simulink model "Template"  (R2021b)
settings: Solver=VariableStepAuto  StartTime=0.0  StopTime=48  RelTol=1e-3
undefined symbols (not defined in the file or in its folder): f650
libraries: simulink x32, slpidlib x1
settings Model: Creator=Admin  LastModifiedBy=Admin
settings SolverCC: AlgebraicLoopSolver=TrustRegion
settings DebuggingCC: SFMachineParentedDataDiag=warning

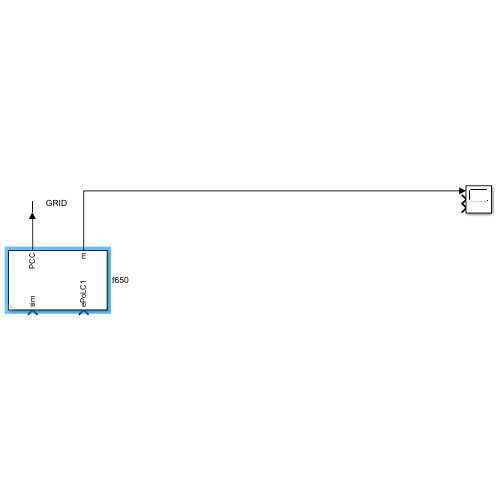
[thumbnail: Simulink's stored preview of the top-level diagram]
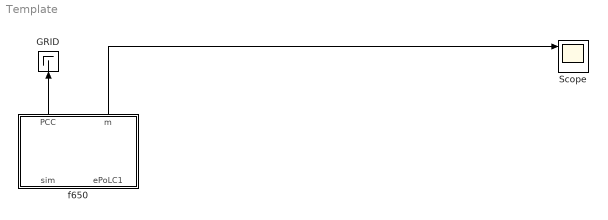
== system Template ==
  GRID : Terminator
  Scope : Scope  NumInputPorts=3
  f650 : Subsystem  mask(Prosumer){sPoLC1sel=External, sPoLC2sel=Disabled, sPoLC3sel=Disabled, sPoLC4sel=Disabled, sPoLC5sel=Disabled, sPoLC6sel=Disabled, sPoLC7sel=Disabled, sPoLC8sel=Disabled, sPoLC9sel=Disabled, sPoLC10sel=Disabled, sPoLC11sel=Disabled, sPoLC12sel=Disabled, sPoLC13sel=Disabled, sPoLC14sel=Disabled, sPoLC15sel=Disabled, sPoLC16sel=Disabled}
      mask prompts: sPoLC1sel "PoLC #1 type"; sPoLC2sel "PoLC #2 type"; sPoLC3sel "PoLC #3 type"; sPoLC4sel "PoLC #4 type"; sPoLC5sel "PoLC #5 type"; sPoLC6sel "PoLC #6 type"; sPoLC7sel "PoLC #7 type"; sPoLC8sel "PoLC #8 type"; sPoLC9sel "PoLC #9 type"; sPoLC10sel "PoLC #10 type"; sPoLC11sel "PoLC #11 type"; sPoLC12sel "PoLC #12 type"; sPoLC13sel "PoLC #13 type"; sPoLC14sel "PoLC #14 type"; sPoLC15sel "PoLC #15 type"; sPoLC16sel "PoLC #16 type"
      mask help:
      | Simplified model of electrical prosumer technological system.
      |
      | V0.1.0
      mask init:
      | % link local generation variables
      | tblk = Simulink.findBlocks(gcb,'Name','base');
      | for i=1:length(tblk)
      |     val = strrep(getfullname(tblk(i)),join([gcs,'/'],''),'');
      |     val = strrep(val,join(['/','base'],''),'');
      |     val = strrep(val,'lPoLC','PoLC');
      |     val = strrep(val,'DEVICES/','');
      |     val = strrep(val,'CONTROLLERS/','');
      |     val = strrep(val,'/','.');
      |     set_param(tblk(i),'OutValues',join([val,'.','l'],''));
      |     set_param(tblk(i),'tsamp',join([val,'.','ST'],''));
      | end
      | 
      | sblk = Simulink.findBlocks(gcb,'Name','noise');
      | for i=1:length(sblk)
      |     val = strrep(getfullname(sblk(i)),join([gcs,'/'],''),'');
      |     val = strrep(val,join(['/','noise'],''),'');
      |     val = strrep(val,'lPoLC','PoLC');
      |     val = strrep(val,'DEVICES/','');
      |     val = strrep(val,'CONTROLLERS/','');
      |     val = strrep(val,'/','.');
      |     set_param(sblk(i),'Cov',join([val,'.','Noise'],''));
      |     set_param(sblk(i),'Ts',join([val,'.','NoiseST'],''));
      |     set_param(sblk(i),'seed',join([val,'.','NoiseSD'],''));
      | end
      mask TypeOptions sPoLC1sel: Disabled | Internal | External
      mask Callback sPoLC1sel: prsmr_functions('1',gcs,gcb);
      mask TypeOptions sPoLC2sel: Disabled | Internal | External
      mask Callback sPoLC2sel: prsmr_functions('2',gcs,gcb)
      mask TypeOptions sPoLC3sel: Disabled | Internal | External
      mask Callback sPoLC3sel: prsmr_functions('3',gcs,gcb)
      mask TypeOptions sPoLC4sel: Disabled | Internal | External
      mask Callback sPoLC4sel: prsmr_functions('4',gcs,gcb)
      mask TypeOptions sPoLC5sel: Disabled | Internal | External
      mask Callback sPoLC5sel: prsmr_functions('5',gcs,gcb)
      mask TypeOptions sPoLC6sel: Disabled | Internal | External
      mask Callback sPoLC6sel: prsmr_functions('6',gcs,gcb)
      mask TypeOptions sPoLC7sel: Disabled | Internal | External
      mask Callback sPoLC7sel: prsmr_functions('7',gcs,gcb)
      mask TypeOptions sPoLC8sel: Disabled | Internal | External
      mask Callback sPoLC8sel: prsmr_functions('8',gcs,gcb)
      mask TypeOptions sPoLC9sel: Disabled | Internal | External
      mask Callback sPoLC9sel: prsmr_functions('9',gcs,gcb)
      mask TypeOptions sPoLC10sel: Disabled | Internal | External
      mask Callback sPoLC10sel: prsmr_functions('10',gcs,gcb)
      mask TypeOptions sPoLC11sel: Disabled | Internal | External
      mask Callback sPoLC11sel: prsmr_functions('11',gcs,gcb)
      mask TypeOptions sPoLC12sel: Disabled | Internal | External
      mask Callback sPoLC12sel: prsmr_functions('12',gcs,gcb)
      mask TypeOptions sPoLC13sel: Disabled | Internal | External
      mask Callback sPoLC13sel: prsmr_functions('13',gcs,gcb)
      mask TypeOptions sPoLC14sel: Disabled | Internal | External
      mask Callback sPoLC14sel: prsmr_functions('14',gcs,gcb)
      mask TypeOptions sPoLC15sel: Disabled | Internal | External
      mask Callback sPoLC15sel: prsmr_functions('15',gcs,gcb)
      mask TypeOptions sPoLC16sel: Disabled | Internal | External
      mask Callback sPoLC16sel: prsmr_functions('16',gcs,gcb)
  wires:
  f650/2(m) -> Scope/1
  f650/1(PCC) -> GRID/1

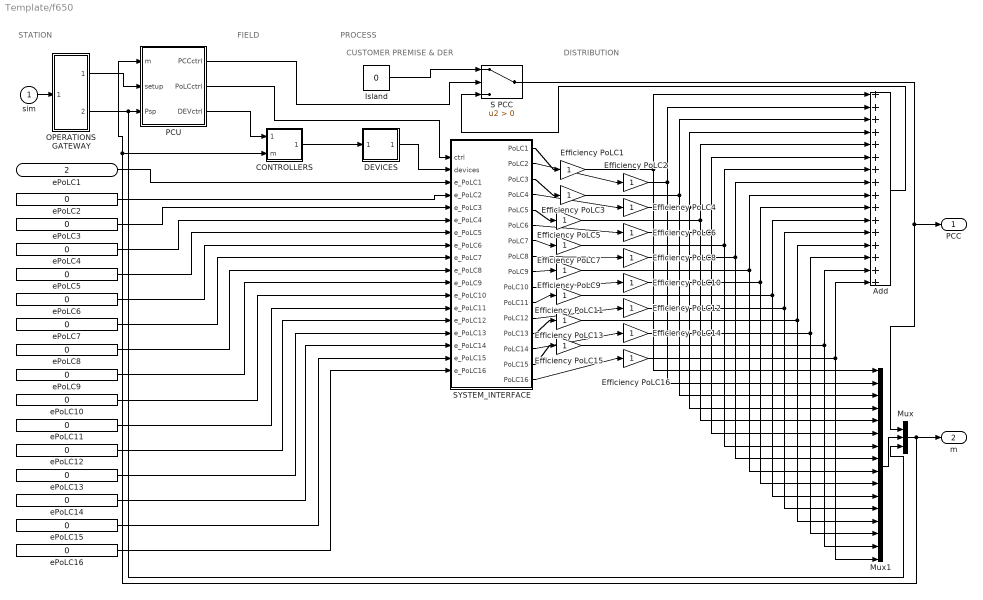
== system Template/f650 ==
  note: PROCESS
  note: STATION
  note: FIELD
  note: DISTRIBUTION
  note: CUSTOMER PREMISE & DER
  sim : Inport
  ePoLC1 : Inport  Port=2
  Add : Sum  Inputs=16
  CONTROLLERS : Subsystem
  DEVICES : Subsystem
  Efficiency PoLC{1..16} (16 alike) : Gain  ParamMin=[0]  ParamMax=[1]
  Island : Constant  Value=0
  Mux : Mux  Inputs=3
  Mux1 : Mux  Inputs=16
  OPERATIONS GATEWAY : Subsystem
  PCU : Subsystem
  S PCC : Switch  Criteria=u2 > Threshold
  SYSTEM_INTERFACE : Subsystem
  ePoLC{2..16} (15 alike) : Constant  Value=0
  PCC : Outport  VectorParamsAs1DForOutWhenUnconnected=off
  m : Outport  Port=2  VectorParamsAs1DForOutWhenUnconnected=off
  wires:
  PCU/1(PCCctrl) -> S PCC/2
  Mux1/1 -> Mux/2
  Island/1 -> S PCC/1
  Mux/1 -> CONTROLLERS/2(m), PCU/1(m), m/1
  S PCC/1 -> Mux/1, PCC/1
  Add/1 -> S PCC/3
  SYSTEM_INTERFACE/2(PoLC2) -> Efficiency PoLC2/1
  SYSTEM_INTERFACE/4(PoLC4) -> Efficiency PoLC4/1
  SYSTEM_INTERFACE/8(PoLC8) -> Efficiency PoLC8/1
  SYSTEM_INTERFACE/5(PoLC5) -> Efficiency PoLC5/1
  SYSTEM_INTERFACE/12(PoLC12) -> Efficiency PoLC12/1
  SYSTEM_INTERFACE/15(PoLC15) -> Efficiency PoLC15/1
  SYSTEM_INTERFACE/6(PoLC6) -> Efficiency PoLC6/1
  SYSTEM_INTERFACE/13(PoLC13) -> Efficiency PoLC13/1
  SYSTEM_INTERFACE/10(PoLC10) -> Efficiency PoLC10/1
  SYSTEM_INTERFACE/3(PoLC3) -> Efficiency PoLC3/1
  SYSTEM_INTERFACE/16(PoLC16) -> Efficiency PoLC16/1
  SYSTEM_INTERFACE/1(PoLC1) -> Efficiency PoLC1/1
  SYSTEM_INTERFACE/11(PoLC11) -> Efficiency PoLC11/1
  SYSTEM_INTERFACE/9(PoLC9) -> Efficiency PoLC9/1
  SYSTEM_INTERFACE/7(PoLC7) -> Efficiency PoLC7/1
  SYSTEM_INTERFACE/14(PoLC14) -> Efficiency PoLC14/1
  ePoLC1/1 -> SYSTEM_INTERFACE/3(e_PoLC1)
  ePoLC2/1 -> SYSTEM_INTERFACE/4(e_PoLC2)
  ePoLC3/1 -> SYSTEM_INTERFACE/5(e_PoLC3)
  ePoLC4/1 -> SYSTEM_INTERFACE/6(e_PoLC4)
  ePoLC5/1 -> SYSTEM_INTERFACE/7(e_PoLC5)
  ePoLC6/1 -> SYSTEM_INTERFACE/8(e_PoLC6)
  ePoLC7/1 -> SYSTEM_INTERFACE/9(e_PoLC7)
  ePoLC8/1 -> SYSTEM_INTERFACE/10(e_PoLC8)
  ePoLC9/1 -> SYSTEM_INTERFACE/11(e_PoLC9)
  ePoLC10/1 -> SYSTEM_INTERFACE/12(e_PoLC10)
  ePoLC11/1 -> SYSTEM_INTERFACE/13(e_PoLC11)
  ePoLC12/1 -> SYSTEM_INTERFACE/14(e_PoLC12)
  ePoLC13/1 -> SYSTEM_INTERFACE/15(e_PoLC13)
  ePoLC14/1 -> SYSTEM_INTERFACE/16(e_PoLC14)
  ePoLC15/1 -> SYSTEM_INTERFACE/17(e_PoLC15)
  ePoLC16/1 -> SYSTEM_INTERFACE/18(e_PoLC16)
  PCU/2(PoLCctrl) -> SYSTEM_INTERFACE/1(ctrl)
  CONTROLLERS/1(dev) -> DEVICES/1(ctrl)
  OPERATIONS GATEWAY/1(setup) -> PCU/2(setup)
  OPERATIONS GATEWAY/2(Psp) -> Mux/3, PCU/3(Psp)
  sim/1 -> OPERATIONS GATEWAY/1(sim)
  PCU/3(DEVctrl) -> CONTROLLERS/1(ctrl)
  DEVICES/1(dev) -> SYSTEM_INTERFACE/2(devices)
  Efficiency PoLC1/1 -> Add/1, Mux1/1
  Efficiency PoLC2/1 -> Add/2, Mux1/2
  Efficiency PoLC3/1 -> Add/3, Mux1/3
  Efficiency PoLC4/1 -> Add/4, Mux1/4
  Efficiency PoLC5/1 -> Add/5, Mux1/5
  Efficiency PoLC6/1 -> Add/6, Mux1/6
  Efficiency PoLC7/1 -> Add/7, Mux1/7
  Efficiency PoLC8/1 -> Add/8, Mux1/8
  Efficiency PoLC9/1 -> Add/9, Mux1/9
  Efficiency PoLC10/1 -> Mux1/10, Add/10
  Efficiency PoLC11/1 -> Add/11, Mux1/11
  Efficiency PoLC12/1 -> Add/12, Mux1/12
  Efficiency PoLC13/1 -> Add/13, Mux1/13
  Efficiency PoLC14/1 -> Add/14, Mux1/14
  Efficiency PoLC15/1 -> Mux1/15, Add/15
  Efficiency PoLC16/1 -> Add/16, Mux1/16

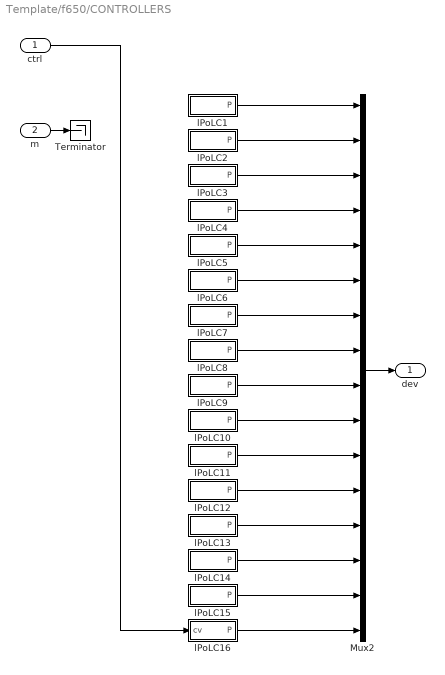
== system Template/f650/CONTROLLERS ==
  ctrl : Inport
  m : Inport  Port=2
  Mux2 : Mux  Inputs=16
  Terminator : Terminator
  lPoLC1 : Subsystem  TreatAsAtomicUnit=on
  lPoLC10 : Subsystem  TreatAsAtomicUnit=on
  lPoLC11 : Subsystem  TreatAsAtomicUnit=on
  lPoLC12 : Subsystem  TreatAsAtomicUnit=on
  lPoLC13 : Subsystem  TreatAsAtomicUnit=on
  lPoLC14 : Subsystem  TreatAsAtomicUnit=on
  lPoLC15 : Subsystem  TreatAsAtomicUnit=on
  lPoLC16 : Subsystem  TreatAsAtomicUnit=on
  lPoLC2 : Subsystem  TreatAsAtomicUnit=on
  lPoLC3 : Subsystem  TreatAsAtomicUnit=on
  lPoLC4 : Subsystem  TreatAsAtomicUnit=on
  lPoLC5 : Subsystem  TreatAsAtomicUnit=on
  lPoLC6 : Subsystem  TreatAsAtomicUnit=on
  lPoLC7 : Subsystem  TreatAsAtomicUnit=on
  lPoLC8 : Subsystem  TreatAsAtomicUnit=on
  lPoLC9 : Subsystem  TreatAsAtomicUnit=on
  dev : Outport  VectorParamsAs1DForOutWhenUnconnected=off
  wires:
  Mux2/1 -> dev/1
  lPoLC1/1(P) -> Mux2/1
  lPoLC2/1(P) -> Mux2/2
  lPoLC16/1(P) -> Mux2/16
  lPoLC3/1(P) -> Mux2/3
  lPoLC4/1(P) -> Mux2/4
  lPoLC5/1(P) -> Mux2/5
  lPoLC6/1(P) -> Mux2/6
  lPoLC7/1(P) -> Mux2/7
  lPoLC8/1(P) -> Mux2/8
  lPoLC9/1(P) -> Mux2/9
  lPoLC10/1(P) -> Mux2/10
  lPoLC11/1(P) -> Mux2/11
  lPoLC12/1(P) -> Mux2/12
  lPoLC13/1(P) -> Mux2/13
  lPoLC14/1(P) -> Mux2/14
  lPoLC15/1(P) -> Mux2/15
  ctrl/1 -> lPoLC16/1(cv)
  m/1 -> Terminator/1

== system Template/f650/DEVICES ==
  ctrl : Inport
  dev : Outport  VectorParamsAs1DForOutWhenUnconnected=off
  wires:
  ctrl/1 -> dev/1

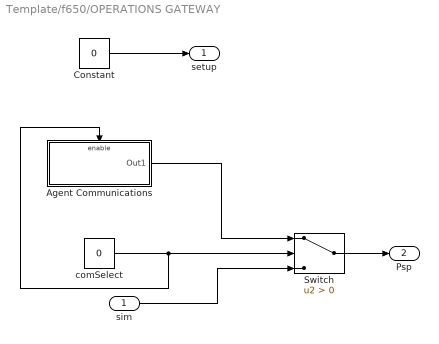
== system Template/f650/OPERATIONS GATEWAY ==
  sim : Inport
  Agent Communications : Subsystem  TreatAsAtomicUnit=on
  Constant : Constant  Value=0
  Switch : Switch  Criteria=u2 > Threshold
  comSelect : Constant  Value=0
  setup : Outport  VectorParamsAs1DForOutWhenUnconnected=off
  Psp : Outport  Port=2  VectorParamsAs1DForOutWhenUnconnected=off
  wires:
  Constant/1 -> setup/1
  sim/1 -> Switch/3
  Switch/1 -> Psp/1
  Agent Communications/1(Out1) -> Switch/1
  comSelect/1 -> Switch/2, Agent Communications/Enable

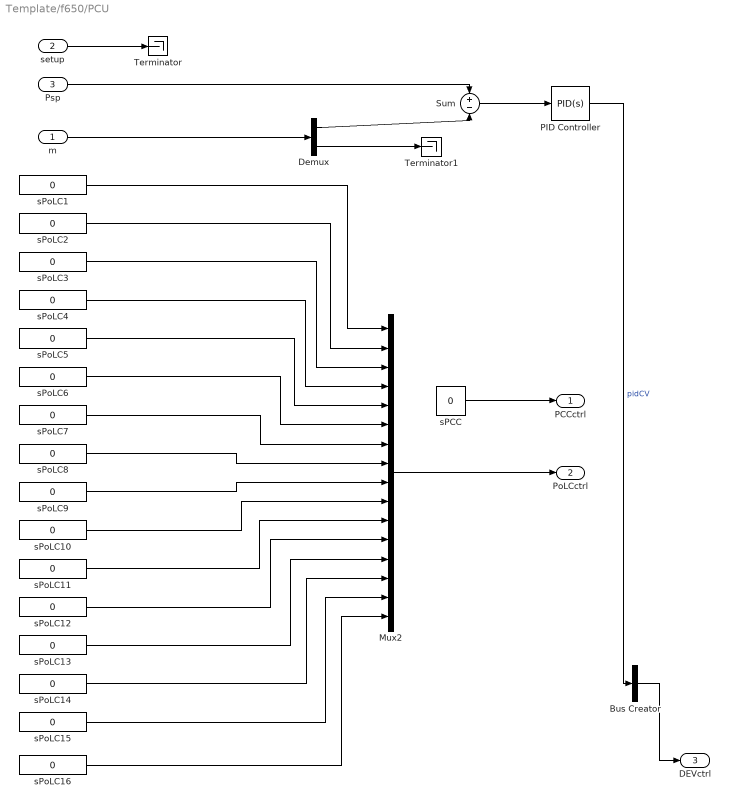
== system Template/f650/PCU ==
  m : Inport
  setup : Inport  Port=2
  Psp : Inport  Port=3
  Bus Creator : BusCreator  Inputs=1
  Demux : Demux  Outputs=[1 -1]
  Mux2 : Mux  Inputs=16
  PID Controller : slpidlib/PID Controller  Controller=PID  Form=Parallel  TimeDomain=Continuous-time  UseExternalTs=off  SampleTime=-1  IntegratorMethod=Forward Euler  FilterMethod=Forward Euler  ControllerParametersSource=internal  P=80  I=20  D=10  UseFilter=on  N=100  TunerSelectOption=Transfer Function Based (PID Tuner App)  InitialConditionSource=internal  InitialConditionForIntegrator=0  InitialConditionForFilter=0  DifferentiatorICPrevScaledInput=0  ExternalReset=none  TrackingMode=off  Kt=1  LimitOutput=off  SatLimitsSource=internal  UpperSaturationLimit=inf  LowerSaturationLimit=-inf  LinearizeAsGain=on  AntiWindupMode=none  Kb=1  POutMin=[]  POutMax=[]  IOutMin=[]  IOutMax=[]  DOutMin=[]  DOutMax=[]  NOutMin=[]  NOutMax=[]  SumOutMin=[]  SumOutMax=[]  SaturationOutMin=[]  SaturationOutMax=[]  PParamMin=[]  PParamMax=[]  IParamMin=[]  IParamMax=[]  DParamMin=[]  DParamMax=[]  NParamMin=[]  NParamMax=[]  KbParamMin=[]  KbParamMax=[]  KtParamMin=[]  KtParamMax=[]  KbOutMin=[]  KbOutMax=[]  KtOutMin=[]  KtOutMax=[]  IntegratorOutMin=[]  IntegratorOutMax=[]  FilterOutMin=[]  FilterOutMax=[]  SumI1OutMin=[]  SumI1OutMax=[]  SumI2OutMin=[]  SumI2OutMax=[]  SumI3OutMin=[]  SumI3OutMax=[]  SumI4OutMin=[]  SumI4OutMax=[]  SumDOutMin=[]  SumDOutMax=[]  DifferentiatorOutMin=[]  DifferentiatorOutMax=[]  FilterDiffOutCoefMin=[]  FilterDiffOutCoefMax=[]  ReciprocalOutMin=[]  ReciprocalOutMax=[]  SumDenOutMin=[]  SumDenOutMax=[]  SumNumOutMin=[]  SumNumOutMax=[]  DivideOutMin=[]  DivideOutMax=[]  UdiffTsProdOutMin=[]  UdiffTsProdOutMax=[]  NTsProdOutMin=[]  NTsProdOutMax=[]  UintegralTsProdOutMin=[]  UintegralTsProdOutMax=[]  UngainTsProdOutMin=[]  UngainTsProdOutMax=[]  IntegratorContinuousStateAttributes=''  IntegratorStateMustResolveToSignalObject=off  IntegratorRTWStateStorageClass=Auto  FilterContinuousStateAttributes=''  FilterStateMustResolveToSignalObject=off  FilterRTWStateStorageClass=Auto  ParallelPVariant=InternalParameters  IdealPVariant=Disabled  IVariant=InternalParameters  DVariant=InternalParameters  IntegratorVariant=Continuous  SatVariant=Disabled  AWVariant=Passthrough  PCopyVariant=Disabled  TRVariant=Disabled  FdbkBlocksVariant=Forward  IdealPFdbkVariant=Disabled  SatFdbkVariant=Disabled  DerivativeFilterVariant=ContFilter  NVariant=InternalParameters  NCopyVariant=Disabled  FilterICVariant=InternalICsFilter  IntegratorICVariant=InternalICs  ExternalResetVariant=Disabled  TRSumVariant=Passthrough  SumFdbkVariant=Disabled  SumVariant=Sum_PID  TsampFilterVariant=InternalTs  TsampNgainVariant=Passthrough  TsampIntegralVariant=Passthrough  ExternalSaturationOutDataTypeStr=Inherit: Same as second input
  Sum : Sum  Inputs=+-
  Terminator : Terminator
  Terminator1 : Terminator
  sPCC : Constant  Value=0
  sPoLC{1..16} (16 alike) : Constant  Value=0
  PCCctrl : Outport  VectorParamsAs1DForOutWhenUnconnected=off
  PoLCctrl : Outport  Port=2  VectorParamsAs1DForOutWhenUnconnected=off
  DEVctrl : Outport  Port=3  VectorParamsAs1DForOutWhenUnconnected=off
  wires:
  sPoLC8/1 -> Mux2/8
  sPoLC11/1 -> Mux2/11
  sPoLC4/1 -> Mux2/4
  sPoLC16/1 -> Mux2/16
  sPoLC14/1 -> Mux2/14
  sPoLC10/1 -> Mux2/10
  sPoLC12/1 -> Mux2/12
  sPoLC1/1 -> Mux2/1
  sPoLC15/1 -> Mux2/15
  sPoLC6/1 -> Mux2/6
  sPoLC13/1 -> Mux2/13
  sPoLC7/1 -> Mux2/7
  sPoLC9/1 -> Mux2/9
  sPoLC2/1 -> Mux2/2
  sPoLC3/1 -> Mux2/3
  sPoLC5/1 -> Mux2/5
  Mux2/1 -> PoLCctrl/1
  sPCC/1 -> PCCctrl/1
  setup/1 -> Terminator/1
  Psp/1 -> Sum/1
  Bus Creator/1 -> DEVctrl/1
  m/1 -> Demux/1
  Demux/1 -> Sum/2
  Sum/1 -> PID Controller/1
  PID Controller/1 -> Bus Creator/1  "pidCV"
  Demux/2 -> Terminator1/1

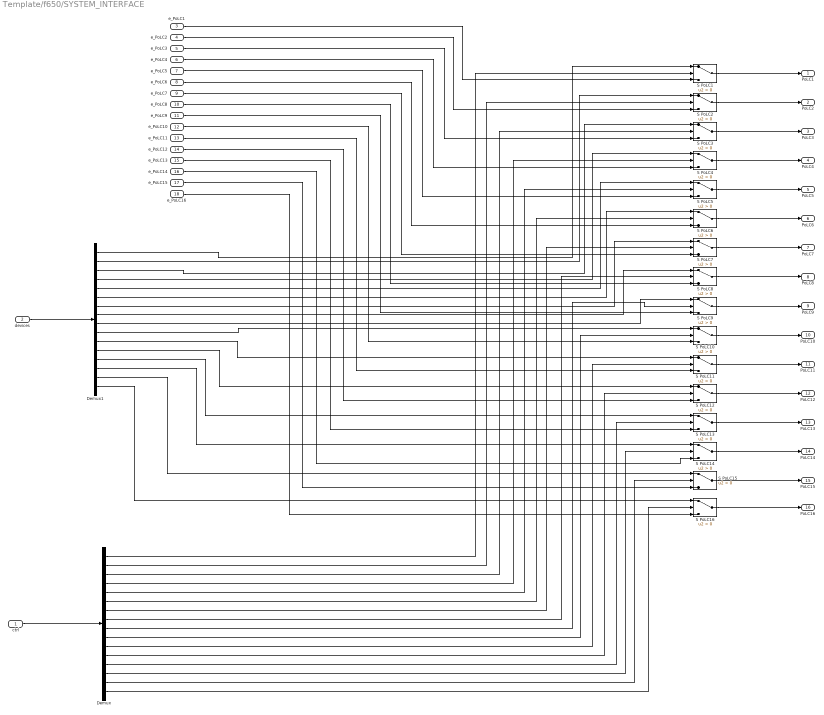
== system Template/f650/SYSTEM_INTERFACE ==
  ctrl : Inport
  devices : Inport  Port=2
  e_PoLC1 : Inport  Port=3
  e_PoLC2 : Inport  Port=4
  e_PoLC3 : Inport  Port=5
  e_PoLC4 : Inport  Port=6
  e_PoLC5 : Inport  Port=7
  e_PoLC6 : Inport  Port=8
  e_PoLC7 : Inport  Port=9
  e_PoLC8 : Inport  Port=10
  e_PoLC9 : Inport  Port=11
  e_PoLC10 : Inport  Port=12
  e_PoLC11 : Inport  Port=13
  e_PoLC12 : Inport  Port=14
  e_PoLC13 : Inport  Port=15
  e_PoLC14 : Inport  Port=16
  e_PoLC15 : Inport  Port=17
  e_PoLC16 : Inport  Port=18
  Demux : Demux  Outputs=16
  Demux1 : Demux  Outputs=16
  S PoLC{1..16} (16 alike) : Switch  Criteria=u2 > Threshold
  PoLC1 : Outport  VectorParamsAs1DForOutWhenUnconnected=off
  PoLC2 : Outport  Port=2  VectorParamsAs1DForOutWhenUnconnected=off
  PoLC3 : Outport  Port=3  VectorParamsAs1DForOutWhenUnconnected=off
  PoLC4 : Outport  Port=4  VectorParamsAs1DForOutWhenUnconnected=off
  PoLC5 : Outport  Port=5  VectorParamsAs1DForOutWhenUnconnected=off
  PoLC6 : Outport  Port=6  VectorParamsAs1DForOutWhenUnconnected=off
  PoLC7 : Outport  Port=7  VectorParamsAs1DForOutWhenUnconnected=off
  PoLC8 : Outport  Port=8  VectorParamsAs1DForOutWhenUnconnected=off
  PoLC9 : Outport  Port=9  VectorParamsAs1DForOutWhenUnconnected=off
  PoLC10 : Outport  Port=10  VectorParamsAs1DForOutWhenUnconnected=off
  PoLC11 : Outport  Port=11  VectorParamsAs1DForOutWhenUnconnected=off
  PoLC12 : Outport  Port=12  VectorParamsAs1DForOutWhenUnconnected=off
  PoLC13 : Outport  Port=13  VectorParamsAs1DForOutWhenUnconnected=off
  PoLC14 : Outport  Port=14  VectorParamsAs1DForOutWhenUnconnected=off
  PoLC15 : Outport  Port=15  VectorParamsAs1DForOutWhenUnconnected=off
  PoLC16 : Outport  Port=16  VectorParamsAs1DForOutWhenUnconnected=off
  wires:
  S PoLC9/1 -> PoLC9/1
  e_PoLC4/1 -> S PoLC4/3
  e_PoLC11/1 -> S PoLC11/3
  S PoLC16/1 -> PoLC16/1
  e_PoLC8/1 -> S PoLC8/3
  S PoLC6/1 -> PoLC6/1
  e_PoLC7/1 -> S PoLC7/3
  S PoLC13/1 -> PoLC13/1
  e_PoLC5/1 -> S PoLC5/3
  S PoLC10/1 -> PoLC10/1
  e_PoLC9/1 -> S PoLC9/3
  e_PoLC12/1 -> S PoLC12/3
  e_PoLC6/1 -> S PoLC6/3
  S PoLC15/1 -> PoLC15/1
  S PoLC1/1 -> PoLC1/1
  S PoLC12/1 -> PoLC12/1
  S PoLC11/1 -> PoLC11/1
  e_PoLC14/1 -> S PoLC14/3
  e_PoLC10/1 -> S PoLC10/3
  S PoLC5/1 -> PoLC5/1
  e_PoLC1/1 -> S PoLC1/3
  e_PoLC15/1 -> S PoLC15/3
  e_PoLC16/1 -> S PoLC16/3
  S PoLC7/1 -> PoLC7/1
  e_PoLC3/1 -> S PoLC3/3
  e_PoLC13/1 -> S PoLC13/3
  S PoLC8/1 -> PoLC8/1
  e_PoLC2/1 -> S PoLC2/3
  S PoLC4/1 -> PoLC4/1
  S PoLC2/1 -> PoLC2/1
  S PoLC14/1 -> PoLC14/1
  S PoLC3/1 -> PoLC3/1
  ctrl/1 -> Demux/1
  Demux/1 -> S PoLC1/2
  Demux/2 -> S PoLC2/2
  Demux/3 -> S PoLC3/2
  Demux/4 -> S PoLC4/2
  Demux/5 -> S PoLC5/2
  Demux/6 -> S PoLC6/2
  Demux/7 -> S PoLC7/2
  Demux/8 -> S PoLC8/2
  Demux/9 -> S PoLC9/2
  Demux/10 -> S PoLC10/2
  Demux/11 -> S PoLC11/2
  Demux/12 -> S PoLC12/2
  Demux/13 -> S PoLC13/2
  Demux/14 -> S PoLC14/2
  Demux/15 -> S PoLC15/2
  Demux/16 -> S PoLC16/2
  devices/1 -> Demux1/1
  Demux1/1 -> S PoLC1/1
  Demux1/2 -> S PoLC2/1
  Demux1/3 -> S PoLC3/1
  Demux1/4 -> S PoLC4/1
  Demux1/5 -> S PoLC5/1
  Demux1/6 -> S PoLC6/1
  Demux1/7 -> S PoLC7/1
  Demux1/8 -> S PoLC8/1
  Demux1/9 -> S PoLC9/1
  Demux1/10 -> S PoLC10/1
  Demux1/11 -> S PoLC11/1
  Demux1/12 -> S PoLC12/1
  Demux1/13 -> S PoLC13/1
  Demux1/14 -> S PoLC14/1
  Demux1/15 -> S PoLC15/1
  Demux1/16 -> S PoLC16/1

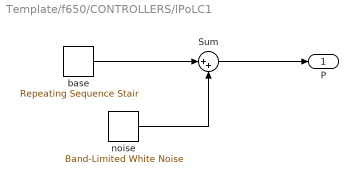
== system Template/f650/CONTROLLERS/lPoLC1 ==
  Sum : Sum  Inputs=|++
  base : simulink/Sources/Repeating Sequence Stair  OutValues=f650.PoLC1.l  tsamp=f650.PoLC1.ST  OutMin=[]  OutMax=[]  OutDataTypeStr=double  OutputDataTypeScalingMode=double  OutDataType=fixdt(0,8)  ConRadixGroup=Best Precision: Vector-wise  OutScaling=2^-12
  noise : simulink/Sources/Band-Limited White Noise  Cov=f650.PoLC1.Noise  Ts=f650.PoLC1.NoiseST  seed=f650.PoLC1.NoiseSD
  P : Outport  VectorParamsAs1DForOutWhenUnconnected=off
  wires:
  Sum/1 -> P/1
  noise/1 -> Sum/2
  base/1 -> Sum/1

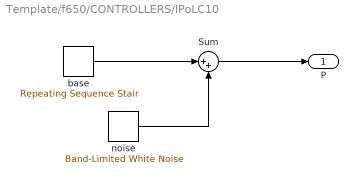
== system Template/f650/CONTROLLERS/lPoLC10 ==
  Sum : Sum  Inputs=|++
  base : simulink/Sources/Repeating Sequence Stair  OutValues=f650.PoLC10.l  tsamp=f650.PoLC10.ST  OutMin=[]  OutMax=[]  OutDataTypeStr=double  OutputDataTypeScalingMode=double  OutDataType=fixdt(0,8)  ConRadixGroup=Best Precision: Vector-wise  OutScaling=2^-12
  noise : simulink/Sources/Band-Limited White Noise  Cov=f650.PoLC10.Noise  Ts=f650.PoLC10.NoiseST  seed=f650.PoLC10.NoiseSD
  P : Outport  VectorParamsAs1DForOutWhenUnconnected=off
  wires:
  Sum/1 -> P/1
  noise/1 -> Sum/2
  base/1 -> Sum/1

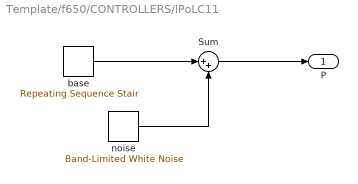
== system Template/f650/CONTROLLERS/lPoLC11 ==
  Sum : Sum  Inputs=|++
  base : simulink/Sources/Repeating Sequence Stair  OutValues=f650.PoLC11.l  tsamp=f650.PoLC11.ST  OutMin=[]  OutMax=[]  OutDataTypeStr=double  OutputDataTypeScalingMode=double  OutDataType=fixdt(0,8)  ConRadixGroup=Best Precision: Vector-wise  OutScaling=2^-12
  noise : simulink/Sources/Band-Limited White Noise  Cov=f650.PoLC11.Noise  Ts=f650.PoLC11.NoiseST  seed=f650.PoLC11.NoiseSD
  P : Outport  VectorParamsAs1DForOutWhenUnconnected=off
  wires:
  Sum/1 -> P/1
  noise/1 -> Sum/2
  base/1 -> Sum/1

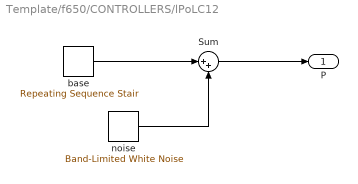
== system Template/f650/CONTROLLERS/lPoLC12 ==
  Sum : Sum  Inputs=|++
  base : simulink/Sources/Repeating Sequence Stair  OutValues=f650.PoLC12.l  tsamp=f650.PoLC12.ST  OutMin=[]  OutMax=[]  OutDataTypeStr=double  OutputDataTypeScalingMode=double  OutDataType=fixdt(0,8)  ConRadixGroup=Best Precision: Vector-wise  OutScaling=2^-12
  noise : simulink/Sources/Band-Limited White Noise  Cov=f650.PoLC12.Noise  Ts=f650.PoLC12.NoiseST  seed=f650.PoLC12.NoiseSD
  P : Outport  VectorParamsAs1DForOutWhenUnconnected=off
  wires:
  Sum/1 -> P/1
  noise/1 -> Sum/2
  base/1 -> Sum/1

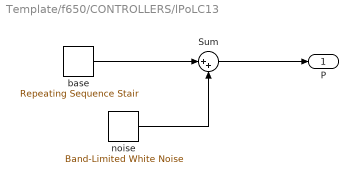
== system Template/f650/CONTROLLERS/lPoLC13 ==
  Sum : Sum  Inputs=|++
  base : simulink/Sources/Repeating Sequence Stair  OutValues=f650.PoLC13.l  tsamp=f650.PoLC13.ST  OutMin=[]  OutMax=[]  OutDataTypeStr=double  OutputDataTypeScalingMode=double  OutDataType=fixdt(0,8)  ConRadixGroup=Best Precision: Vector-wise  OutScaling=2^-12
  noise : simulink/Sources/Band-Limited White Noise  Cov=f650.PoLC13.Noise  Ts=f650.PoLC13.NoiseST  seed=f650.PoLC13.NoiseSD
  P : Outport  VectorParamsAs1DForOutWhenUnconnected=off
  wires:
  Sum/1 -> P/1
  noise/1 -> Sum/2
  base/1 -> Sum/1

== system Template/f650/CONTROLLERS/lPoLC14 ==
  Sum : Sum  Inputs=|++
  base : simulink/Sources/Repeating Sequence Stair  OutValues=f650.PoLC14.l  tsamp=f650.PoLC14.ST  OutMin=[]  OutMax=[]  OutDataTypeStr=double  OutputDataTypeScalingMode=double  OutDataType=fixdt(0,8)  ConRadixGroup=Best Precision: Vector-wise  OutScaling=2^-12
  noise : simulink/Sources/Band-Limited White Noise  Cov=f650.PoLC14.Noise  Ts=f650.PoLC14.NoiseST  seed=f650.PoLC14.NoiseSD
  P : Outport  VectorParamsAs1DForOutWhenUnconnected=off
  wires:
  Sum/1 -> P/1
  noise/1 -> Sum/2
  base/1 -> Sum/1

== system Template/f650/CONTROLLERS/lPoLC15 ==
  Sum : Sum  Inputs=|++
  base : simulink/Sources/Repeating Sequence Stair  OutValues=f650.PoLC15.l  tsamp=f650.PoLC15.ST  OutMin=[]  OutMax=[]  OutDataTypeStr=double  OutputDataTypeScalingMode=double  OutDataType=fixdt(0,8)  ConRadixGroup=Best Precision: Vector-wise  OutScaling=2^-12
  noise : simulink/Sources/Band-Limited White Noise  Cov=f650.PoLC15.Noise  Ts=f650.PoLC15.NoiseST  seed=f650.PoLC15.NoiseSD
  P : Outport  VectorParamsAs1DForOutWhenUnconnected=off
  wires:
  Sum/1 -> P/1
  noise/1 -> Sum/2
  base/1 -> Sum/1

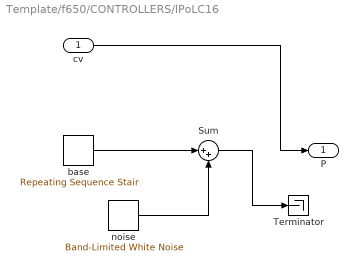
== system Template/f650/CONTROLLERS/lPoLC16 ==
  cv : Inport
  Sum : Sum  Inputs=|++
  Terminator : Terminator
  base : simulink/Sources/Repeating Sequence Stair  OutValues=f650.PoLC16.l  tsamp=f650.PoLC16.ST  OutMin=[]  OutMax=[]  OutDataTypeStr=double  OutputDataTypeScalingMode=double  OutDataType=fixdt(0,8)  ConRadixGroup=Best Precision: Vector-wise  OutScaling=2^-12
  noise : simulink/Sources/Band-Limited White Noise  Cov=f650.PoLC16.Noise  Ts=f650.PoLC16.NoiseST  seed=f650.PoLC16.NoiseSD
  P : Outport  VectorParamsAs1DForOutWhenUnconnected=off
  wires:
  Sum/1 -> Terminator/1
  noise/1 -> Sum/2
  base/1 -> Sum/1
  cv/1 -> P/1

== system Template/f650/CONTROLLERS/lPoLC2 ==
  Sum : Sum  Inputs=|++
  base : simulink/Sources/Repeating Sequence Stair  OutValues=f650.PoLC2.l  tsamp=f650.PoLC2.ST  OutMin=[]  OutMax=[]  OutDataTypeStr=double  OutputDataTypeScalingMode=double  OutDataType=fixdt(0,8)  ConRadixGroup=Best Precision: Vector-wise  OutScaling=2^-12
  noise : simulink/Sources/Band-Limited White Noise  Cov=f650.PoLC2.Noise  Ts=f650.PoLC2.NoiseST  seed=f650.PoLC2.NoiseSD
  P : Outport  VectorParamsAs1DForOutWhenUnconnected=off
  wires:
  Sum/1 -> P/1
  noise/1 -> Sum/2
  base/1 -> Sum/1

== system Template/f650/CONTROLLERS/lPoLC3 ==
  Sum : Sum  Inputs=|++
  base : simulink/Sources/Repeating Sequence Stair  OutValues=f650.PoLC3.l  tsamp=f650.PoLC3.ST  OutMin=[]  OutMax=[]  OutDataTypeStr=double  OutputDataTypeScalingMode=double  OutDataType=fixdt(0,8)  ConRadixGroup=Best Precision: Vector-wise  OutScaling=2^-12
  noise : simulink/Sources/Band-Limited White Noise  Cov=f650.PoLC3.Noise  Ts=f650.PoLC3.NoiseST  seed=f650.PoLC3.NoiseSD
  P : Outport  VectorParamsAs1DForOutWhenUnconnected=off
  wires:
  Sum/1 -> P/1
  noise/1 -> Sum/2
  base/1 -> Sum/1

== system Template/f650/CONTROLLERS/lPoLC4 ==
  Sum : Sum  Inputs=|++
  base : simulink/Sources/Repeating Sequence Stair  OutValues=f650.PoLC4.l  tsamp=f650.PoLC4.ST  OutMin=[]  OutMax=[]  OutDataTypeStr=double  OutputDataTypeScalingMode=double  OutDataType=fixdt(0,8)  ConRadixGroup=Best Precision: Vector-wise  OutScaling=2^-12
  noise : simulink/Sources/Band-Limited White Noise  Cov=f650.PoLC4.Noise  Ts=f650.PoLC4.NoiseST  seed=f650.PoLC4.NoiseSD
  P : Outport  VectorParamsAs1DForOutWhenUnconnected=off
  wires:
  Sum/1 -> P/1
  noise/1 -> Sum/2
  base/1 -> Sum/1

== system Template/f650/CONTROLLERS/lPoLC5 ==
  Sum : Sum  Inputs=|++
  base : simulink/Sources/Repeating Sequence Stair  OutValues=f650.PoLC5.l  tsamp=f650.PoLC5.ST  OutMin=[]  OutMax=[]  OutDataTypeStr=double  OutputDataTypeScalingMode=double  OutDataType=fixdt(0,8)  ConRadixGroup=Best Precision: Vector-wise  OutScaling=2^-12
  noise : simulink/Sources/Band-Limited White Noise  Cov=f650.PoLC5.Noise  Ts=f650.PoLC5.NoiseST  seed=f650.PoLC5.NoiseSD
  P : Outport  VectorParamsAs1DForOutWhenUnconnected=off
  wires:
  Sum/1 -> P/1
  noise/1 -> Sum/2
  base/1 -> Sum/1

== system Template/f650/CONTROLLERS/lPoLC6 ==
  Sum : Sum  Inputs=|++
  base : simulink/Sources/Repeating Sequence Stair  OutValues=f650.PoLC6.l  tsamp=f650.PoLC6.ST  OutMin=[]  OutMax=[]  OutDataTypeStr=double  OutputDataTypeScalingMode=double  OutDataType=fixdt(0,8)  ConRadixGroup=Best Precision: Vector-wise  OutScaling=2^-12
  noise : simulink/Sources/Band-Limited White Noise  Cov=f650.PoLC6.Noise  Ts=f650.PoLC6.NoiseST  seed=f650.PoLC6.NoiseSD
  P : Outport  VectorParamsAs1DForOutWhenUnconnected=off
  wires:
  Sum/1 -> P/1
  noise/1 -> Sum/2
  base/1 -> Sum/1

== system Template/f650/CONTROLLERS/lPoLC7 ==
  Sum : Sum  Inputs=|++
  base : simulink/Sources/Repeating Sequence Stair  OutValues=f650.PoLC7.l  tsamp=f650.PoLC7.ST  OutMin=[]  OutMax=[]  OutDataTypeStr=double  OutputDataTypeScalingMode=double  OutDataType=fixdt(0,8)  ConRadixGroup=Best Precision: Vector-wise  OutScaling=2^-12
  noise : simulink/Sources/Band-Limited White Noise  Cov=f650.PoLC7.Noise  Ts=f650.PoLC7.NoiseST  seed=f650.PoLC7.NoiseSD
  P : Outport  VectorParamsAs1DForOutWhenUnconnected=off
  wires:
  Sum/1 -> P/1
  noise/1 -> Sum/2
  base/1 -> Sum/1

== system Template/f650/CONTROLLERS/lPoLC8 ==
  Sum : Sum  Inputs=|++
  base : simulink/Sources/Repeating Sequence Stair  OutValues=f650.PoLC8.l  tsamp=f650.PoLC8.ST  OutMin=[]  OutMax=[]  OutDataTypeStr=double  OutputDataTypeScalingMode=double  OutDataType=fixdt(0,8)  ConRadixGroup=Best Precision: Vector-wise  OutScaling=2^-12
  noise : simulink/Sources/Band-Limited White Noise  Cov=f650.PoLC8.Noise  Ts=f650.PoLC8.NoiseST  seed=f650.PoLC8.NoiseSD
  P : Outport  VectorParamsAs1DForOutWhenUnconnected=off
  wires:
  Sum/1 -> P/1
  noise/1 -> Sum/2
  base/1 -> Sum/1

== system Template/f650/CONTROLLERS/lPoLC9 ==
  Sum : Sum  Inputs=|++
  base : simulink/Sources/Repeating Sequence Stair  OutValues=f650.PoLC9.l  tsamp=f650.PoLC9.ST  OutMin=[]  OutMax=[]  OutDataTypeStr=double  OutputDataTypeScalingMode=double  OutDataType=fixdt(0,8)  ConRadixGroup=Best Precision: Vector-wise  OutScaling=2^-12
  noise : simulink/Sources/Band-Limited White Noise  Cov=f650.PoLC9.Noise  Ts=f650.PoLC9.NoiseST  seed=f650.PoLC9.NoiseSD
  P : Outport  VectorParamsAs1DForOutWhenUnconnected=off
  wires:
  Sum/1 -> P/1
  noise/1 -> Sum/2
  base/1 -> Sum/1

== system Template/f650/OPERATIONS GATEWAY/Agent Communications ==
  Enable : EnablePort
  Constant : Constant  Value=0
  Out1 : Outport  VectorParamsAs1DForOutWhenUnconnected=off
  wires:
  Constant/1 -> Out1/1
